simulink model "Robot_moding"  (R2019a)
settings: Solver=FixedStepDiscrete  StartTime=0.0  StopTime=10.0  FixedStep=0.1  RelTol=1e-3  EnableMultiTasking=on
settings Model: Creator=YUMU  LastModifiedBy=YUMU
settings SolverCC: AutoInsertRateTranBlk=on
settings DataIOCC: LimitDataPoints=on
settings OptimizationCC: LifeSpan=inf
settings DebuggingCC: AllowSymbolicDim=off  SFUnexpectedBacktrackingDiag=warning  SFNoUnconditionalDefaultTransitionDiag=warning  SFExecutionAtInitializationDiag=none  ArithmeticOperatorsInVariantConditions=warning
settings SFSimCC: SimUseLocalCustomCode=off
settings RTWCC: RTWUseLocalCustomCode=off
settings CodeAppCC: StateflowObjectComments=on
settings GRTTargetCC: TargetLangStandard=C89/C90 (ANSI)  GeneratePreprocessorConditionals=Disable all
settings ConfigComp: CovMetricSettings=dw  CovHtmlReporting=on  CovSaveCumulativeToWorkspaceVar=on  CovSaveSingleToWorkspaceVar=on  CovShowResultsExplorer=off  CovExternalEMLEnable=off  CovSFcnEnable=off

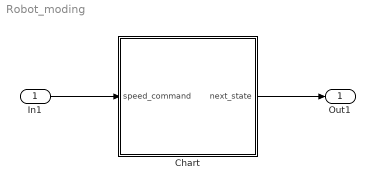
== system Robot_moding ==
  In1 : Inport  OutDataTypeStr=uint8
  Chart : Stateflow chart  TreatAsAtomicUnit=on
  Out1 : Outport  OutDataTypeStr=uint8
  wires:
  In1/1 -> Chart/1(speed_command)
  Chart/1(next_state) -> Out1/1

== stateflow chart Robot_moding/Chart ==
  settings: stateMachineType=MEALY_MACHINE
  state stop_state
  state fast_running
  state slow_running
  (default) -> stop_state
  fast_running -> stop_state [order 1] : [speed_command==0]{next_state=0}
  slow_running -> stop_state [order 2] : [speed_command==0]{next_state=0}
  stop_state -> slow_running [order 2] : [speed_command==1]{next_state=1}
  stop_state -> fast_running [order 1] : [speed_command==2]{next_state=2}
  fast_running -> slow_running [order 2] : [speed_command==1]{next_state=1}
  slow_running -> fast_running [order 1] : [speed_command==2]{next_state=2}
  data: next_state output uint8; speed_command input uint8
